simulink library "exampleMicrogridLibrary"  (R2018a)
settings: Solver=VariableStepAuto  StartTime=0.0  StopTime=10.0  RelTol=1e-3
undefined symbols (not defined in the file or in its folder): BR, D1, Delta, DiscIntNeverNeededParam, Fn, Fnom, gcbh, Ion, kv, Lithium, Ls, Rs, sps_rtmsupport, Ts, Ts_Control, Vn, Vrms
libraries: powerlib x80, simulink x29, powerlib_meascontrol x28, sps_avr x5, spsDieselMotorModel x3, electricdrivelib x2, re_lib x1
(part 2 of 5)

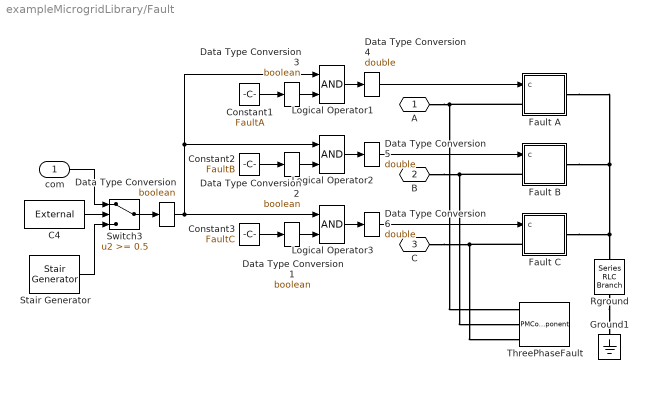
== system exampleMicrogridLibrary/Fault  ==
  com : Inport
  C4 : Constant  Value=External
  Constant1 : Constant  Value=FaultA
  Constant2 : Constant  Value=FaultB
  Constant3 : Constant  Value=FaultC
  Data Type Conversion{,1..3} (4 alike) : DataTypeConversion  OutDataTypeStr=boolean  SaturateOnIntegerOverflow=on  RndMeth=Zero
  Data Type Conversion4 : DataTypeConversion  OutDataTypeStr=double  SaturateOnIntegerOverflow=on  RndMeth=Zero
  Data Type Conversion5 : DataTypeConversion  OutDataTypeStr=double  SaturateOnIntegerOverflow=on  RndMeth=Zero
  Data Type Conversion6 : DataTypeConversion  OutDataTypeStr=double  SaturateOnIntegerOverflow=on  RndMeth=Zero
  Fault A : Subsystem  DialogController=POWERSYS.PowerSysDialog  LoadFcn=sps_rtmsupport('LoadFcn',gcbh);  StartFcn=sps_rtmsupport('StartFcn',gcbh);  StopFcn=sps_rtmsupport('StopFcn',gcbh);  mask(Breaker){InitialState=InitialStates(1)*FaultA, SwitchingTimes=[ 1/60  5/60 ], External=on, BreakerResistance=FaultResistance, SnubberResistance=SnubberResistance, SnubberCapacitance=SnubberCapacitance, Measurements=Branch current, MoreParameters=off, NoBreakLoop=off}
      mask prompts: InitialState "Initial status:"; SwitchingTimes "Switching times (s):"; BreakerResistance "Breaker resistance Ron (Ohm):"; SnubberResistance "Snubber resistance Rs (Ohm):"; SnubberCapacitance "Snubber capacitance Cs (F):"; MoreParameters "obsolete"; NoBreakLoop "Enable zero crossing detection (create an algebraic loop)"
      mask help: Implements a circuit breaker. When the external switching time option is selected, a Simulink logical signal is used to control the breaker operation.
      mask init:
      | block = gcb;
      | [WantBlockChoice,Ts,X,Y,BR,Ron] = powericon('SwitchesInit','Breaker',block,SnubberResistance,SnubberCapacitance,BreakerResistance,InitialState,SwitchingTimes,External);
      | %powericon('SetInternalModels','set',block,WantBlockChoice);
      settings: CopyFcn=sps_rtmsupport('CopyFcn',gcbh); powericon('SwitchesCopyFcn','Breaker',gcb)  DeleteFcn=sps_rtmsupport('DeleteFcn',gcbh);  UndoDeleteFcn=sps_rtmsupport('UndoDeleteFcn',gcbh);  ModelCloseFcn=sps_rtmsupport('ModelCloseFcn',gcbh);  PreSaveFcn=sps_rtmsupport('PreSaveFcn',gcbh);  PostSaveFcn=sps_rtmsupport('PostSaveFcn',gcbh);  NameChangeFcn=sps_rtmsupport('NameChangeFcn',gcbh);  PreCopyFcn=sps_rtmsupport('PreCopyFcn',gcbh);  OpenFcn=sps_rtmsupport('OpenFcn',gcbh, [3 7 8 9]);  CloseFcn=sps_rtmsupport('CloseFcn',gcbh);  PreDeleteFcn=sps_rtmsupport('PreDeleteFcn',gcbh);
      mask Help: helpview(psbhelp);
      mask Callback External: powericon('BreakerCback',gcb);
      mask Callback BreakerResistance: powericon('SwitchesEnables',gcb,'Breaker');
      mask TypeOptions Measurements: None | Branch voltage | Branch current | Branch voltage and current
      mask Display: % plot(X.p1,Y.p1,X.p2,Y.p2,X.p3,Y.p3,X.p4,Y.p4,X.p5,Y.p5,X.p6,Y.p6)
  Fault B : Subsystem  DialogController=POWERSYS.PowerSysDialog  LoadFcn=sps_rtmsupport('LoadFcn',gcbh);  StartFcn=sps_rtmsupport('StartFcn',gcbh);  StopFcn=sps_rtmsupport('StopFcn',gcbh);  mask(Breaker){InitialState=InitialStates(1)*FaultB, SwitchingTimes=[ 1/60  5/60 ], External=on, BreakerResistance=FaultResistance, SnubberResistance=SnubberResistance, SnubberCapacitance=SnubberCapacitance, Measurements=Branch current, MoreParameters=off, NoBreakLoop=off}
      mask prompts: InitialState "Initial status:"; SwitchingTimes "Switching times (s):"; BreakerResistance "Breaker resistance Ron (Ohm):"; SnubberResistance "Snubber resistance Rs (Ohm):"; SnubberCapacitance "Snubber capacitance Cs (F):"; MoreParameters "obsolete"; NoBreakLoop "Enable zero crossing detection (create an algebraic loop)"
      mask help: Implements a circuit breaker. When the external switching time option is selected, a Simulink logical signal is used to control the breaker operation.
      mask init: same as exampleMicrogridLibrary/Fault /Fault A
      settings: CopyFcn=sps_rtmsupport('CopyFcn',gcbh); powericon('SwitchesCopyFcn','Breaker',gcb)  DeleteFcn=sps_rtmsupport('DeleteFcn',gcbh);  UndoDeleteFcn=sps_rtmsupport('UndoDeleteFcn',gcbh);  ModelCloseFcn=sps_rtmsupport('ModelCloseFcn',gcbh);  PreSaveFcn=sps_rtmsupport('PreSaveFcn',gcbh);  PostSaveFcn=sps_rtmsupport('PostSaveFcn',gcbh);  NameChangeFcn=sps_rtmsupport('NameChangeFcn',gcbh);  PreCopyFcn=sps_rtmsupport('PreCopyFcn',gcbh);  OpenFcn=sps_rtmsupport('OpenFcn',gcbh, [3 7 8 9]);  CloseFcn=sps_rtmsupport('CloseFcn',gcbh);  PreDeleteFcn=sps_rtmsupport('PreDeleteFcn',gcbh);
      mask Help: helpview(psbhelp);
      mask Callback External: powericon('BreakerCback',gcb);
      mask Callback BreakerResistance: powericon('SwitchesEnables',gcb,'Breaker');
      mask TypeOptions Measurements: None | Branch voltage | Branch current | Branch voltage and current
      mask Display: % plot(X.p1,Y.p1,X.p2,Y.p2,X.p3,Y.p3,X.p4,Y.p4,X.p5,Y.p5,X.p6,Y.p6)
  Fault C : Subsystem  DialogController=POWERSYS.PowerSysDialog  LoadFcn=sps_rtmsupport('LoadFcn',gcbh);  StartFcn=sps_rtmsupport('StartFcn',gcbh);  StopFcn=sps_rtmsupport('StopFcn',gcbh);  mask(Breaker){InitialState=InitialStates(1)*FaultC, SwitchingTimes=[ 1/60  5/60 ], External=on, BreakerResistance=FaultResistance, SnubberResistance=SnubberResistance, SnubberCapacitance=SnubberCapacitance, Measurements=Branch current, MoreParameters=off, NoBreakLoop=off}
      mask prompts: InitialState "Initial status:"; SwitchingTimes "Switching times (s):"; BreakerResistance "Breaker resistance Ron (Ohm):"; SnubberResistance "Snubber resistance Rs (Ohm):"; SnubberCapacitance "Snubber capacitance Cs (F):"; MoreParameters "obsolete"; NoBreakLoop "Enable zero crossing detection (create an algebraic loop)"
      mask help: Implements a circuit breaker. When the external switching time option is selected, a Simulink logical signal is used to control the breaker operation.
      mask init: same as exampleMicrogridLibrary/Fault /Fault A
      settings: CopyFcn=sps_rtmsupport('CopyFcn',gcbh); powericon('SwitchesCopyFcn','Breaker',gcb)  DeleteFcn=sps_rtmsupport('DeleteFcn',gcbh);  UndoDeleteFcn=sps_rtmsupport('UndoDeleteFcn',gcbh);  ModelCloseFcn=sps_rtmsupport('ModelCloseFcn',gcbh);  PreSaveFcn=sps_rtmsupport('PreSaveFcn',gcbh);  PostSaveFcn=sps_rtmsupport('PostSaveFcn',gcbh);  NameChangeFcn=sps_rtmsupport('NameChangeFcn',gcbh);  PreCopyFcn=sps_rtmsupport('PreCopyFcn',gcbh);  OpenFcn=sps_rtmsupport('OpenFcn',gcbh, [3 7 8 9]);  CloseFcn=sps_rtmsupport('CloseFcn',gcbh);  PreDeleteFcn=sps_rtmsupport('PreDeleteFcn',gcbh);
      mask Help: helpview(psbhelp);
      mask Callback External: powericon('BreakerCback',gcb);
      mask Callback BreakerResistance: powericon('SwitchesEnables',gcb,'Breaker');
      mask TypeOptions Measurements: None | Branch voltage | Branch current | Branch voltage and current
      mask Display: % plot(X.p1,Y.p1,X.p2,Y.p2,X.p3,Y.p3,X.p4,Y.p4,X.p5,Y.p5,X.p6,Y.p6)
  Ground1 : powerlib/Elements/Ground  LConnTagsString=a
  Logical Operator1 : Logic
  Logical Operator2 : Logic
  Logical Operator3 : Logic
  Rground : powerlib/Elements/Series RLC Branch  LConnTagsString=__new0  RConnTagsString=__new0  BranchType=R  Resistance=GroundResistance  Inductance=0  SetiL0=off  InitialCurrent=0  Capacitance=inf  Setx0=off  InitialVoltage=0  Measurements=None
  Stair Generator : powerlib_meascontrol/Pulse & Signal Generators/Stair Generator  t=SwitchTimes  e=SwitchStatus  Ts=Ts
      settings: SourceProductName=Simscape Power Systems
  Switch3 : Switch  Threshold=0.5  ZeroCross=off  InputSameDT=on
  ThreePhaseFault : PMComponent  PhysicalDomain=powersysdomain  LeftPortType=p1  RightPortType=p1  LConnTagsString=A|B|C  mask(InnerPowersysBlock){}
  A : PMIOPort  Side=Left
  B : PMIOPort  Port=2  Side=Left
  C : PMIOPort  Port=3  Side=Left
  wires:
  Data Type Conversion6/1 -> Fault C/1(c)
  Data Type Conversion5/1 -> Fault B/1(c)
  Data Type Conversion4/1 -> Fault A/1(c)
  Logical Operator3/1 -> Data Type Conversion6/1
  Logical Operator2/1 -> Data Type Conversion5/1
  Logical Operator1/1 -> Data Type Conversion4/1
  Data Type Conversion3/1 -> Logical Operator1/2
  Constant1/1 -> Data Type Conversion3/1
  Data Type Conversion2/1 -> Logical Operator2/2
  Constant2/1 -> Data Type Conversion2/1
  Data Type Conversion1/1 -> Logical Operator3/2
  Constant3/1 -> Data Type Conversion1/1
  Data Type Conversion/1 -> Logical Operator1/1, Logical Operator2/1, Logical Operator3/1
  Switch3/1 -> Data Type Conversion/1
  C4/1 -> Switch3/2
  Stair Generator/1 -> Switch3/3
  com/1 -> Switch3/1
  connections:
  Fault B/RConn1 -- Fault A/RConn1 -- Fault C/RConn1 -- Rground/LConn1
  C/RConn1 -- Fault C/LConn1 -- ThreePhaseFault/LConn3
  B/RConn1 -- Fault B/LConn1 -- ThreePhaseFault/LConn2
  A/RConn1 -- Fault A/LConn1 -- ThreePhaseFault/LConn1
  Rground/RConn1 -- Ground1/LConn1

== system exampleMicrogridLibrary/Grid-Connected Battery (EMT with Simple Controls) ==
  PQref : Inport  SampleTime=Ts_Control
  Battery : electricdrivelib/Extra Sources/Battery  BatType=Lithium-Ion  ShowTempParam=off  ThermalPreset=no  ShowAgeParam=off  NomV=Vnom_dc  NomQ=Bcap  SOC=75  Batt_Tr=30  PresetModel=on  MaxQ=500  MinV=360  FullV=558.7138  Dis_rate=217.3913  R=0.0096  Normal_OP=452.1739  expZone="[518.5852      24.56522]"  current=[6.5 13 32.5]  Units=Time  Tci=20  NomT=25  T2=0  MaxQ2=2.208  FullV2=3.45  Normal_OP2=2.8  expZone2="[3.22        0.23]"  Rca=0.6  ti=1000  Dp=0  Neq0=0  Tsim=1e6  Ta1=25  Qeol=5.4*0.9  Reol=0.013333*1.2  Char_age=[2.3478, 3]  Dis_age=[2.3478, 10]  N1=1500  N2=10500  N3=1000  N4=1400  Ta2=45  N5=950
  Battery Controller : Subsystem  SystemSampleTime=Ts
  Bus Selector : BusSelector  OutputSignals=Vabc,Iabc
  DC Link : Subsystem
  Grid Inverter : Subsystem
  Inverter Control : Subsystem
  Measures : Subsystem
  Rate Transition2 : RateTransition  OutPortSampleTime=Ts_Control
  A : PMIOPort  Side=Right
  B : PMIOPort  Port=2  Side=Right
  C : PMIOPort  Port=3  Side=Right
  m : Outport
  wires:
  PQref/1 -> Battery Controller/2(PQref)
  Rate Transition2/1 -> Battery Controller/1(m), Bus Selector/1
  Inverter Control/1(Uref) -> Grid Inverter/1(Uref)
  Bus Selector/1 -> Inverter Control/1(Vabc_prim)  "<Vabc>"
  Bus Selector/2 -> Inverter Control/2(Iabc_prim)  "<Iabc>"
  Grid Inverter/1(m) -> [m_inv]
  [m_inv] -> Measures/1(Grid)
  [m_batt] -> Measures/2(Battery)
  Measures/1(m) -> m/1
  Battery/1 -> [m_batt]
  [m_inv] -> Rate Transition2/1
  Battery Controller/1(Idq_ref) -> Inverter Control/3(Idq_ref)
  connections:
  Battery/LConn1 -- DC Link/LConn1
  Battery/LConn2 -- DC Link/LConn2
  Grid Inverter/LConn3 -- DC Link/RConn3
  A/RConn1 -- Grid Inverter/RConn1
  B/RConn1 -- Grid Inverter/RConn2
  C/RConn1 -- Grid Inverter/RConn3
  Grid Inverter/LConn1 -- DC Link/RConn1
  DC Link/RConn2 -- Grid Inverter/LConn2

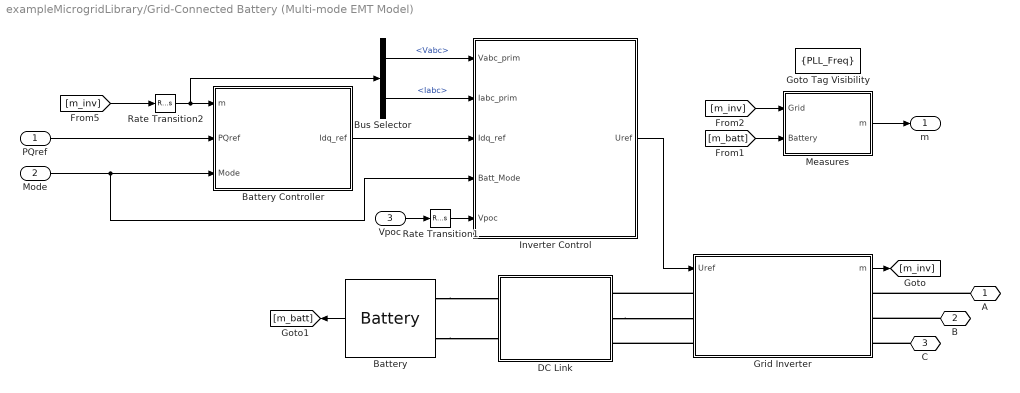
== system exampleMicrogridLibrary/Grid-Connected Battery (Multi-mode EMT Model) ==
  PQref : Inport  SampleTime=Ts_Control
  Mode : Inport  Port=2
  Vpoc : Inport  Port=3
  Battery : electricdrivelib/Extra Sources/Battery  BatType=Lithium-Ion  ShowTempParam=off  ThermalPreset=no  ShowAgeParam=off  NomV=Vnom_dc  NomQ=Bcap  SOC=75  Batt_Tr=30  PresetModel=on  MaxQ=500  MinV=360  FullV=558.7138  Dis_rate=217.3913  R=0.0096  Normal_OP=452.1739  expZone="[518.5852      24.56522]"  current=[6.5 13 32.5]  Units=Time  Tci=20  NomT=25  T2=0  MaxQ2=2.208  FullV2=3.45  Normal_OP2=2.8  expZone2="[3.22        0.23]"  Rca=0.6  ti=1000  Dp=0  Neq0=0  Tsim=1e6  Ta1=25  Qeol=5.4*0.9  Reol=0.013333*1.2  Char_age=[2.3478, 3]  Dis_age=[2.3478, 10]  N1=1500  N2=10500  N3=1000  N4=1400  Ta2=45  N5=950
  Battery Controller : Subsystem  SystemSampleTime=Ts
  Bus Selector : BusSelector  OutputSignals=Vabc,Iabc
  DC Link : Subsystem
  Goto Tag Visibility : GotoTagVisibility  GotoTag=PLL_Freq
  Grid Inverter : Subsystem
  Inverter Control : Subsystem
  Measures : Subsystem
  Rate Transition1 : RateTransition  OutPortSampleTime=Ts_Control
  Rate Transition2 : RateTransition  OutPortSampleTime=Ts_Control
  A : PMIOPort  Side=Right
  B : PMIOPort  Port=2  Side=Right
  C : PMIOPort  Port=3  Side=Right
  m : Outport
  wires:
  Battery Controller/1(Idq_ref) -> Inverter Control/3(Idq_ref)
  [m_inv] -> Rate Transition2/1
  Battery/1 -> [m_batt]
  Measures/1(m) -> m/1
  [m_batt] -> Measures/2(Battery)
  [m_inv] -> Measures/1(Grid)
  Grid Inverter/1(m) -> [m_inv]
  Bus Selector/2 -> Inverter Control/2(Iabc_prim)  "<Iabc>"
  Bus Selector/1 -> Inverter Control/1(Vabc_prim)  "<Vabc>"
  Inverter Control/1(Uref) -> Grid Inverter/1(Uref)
  Rate Transition2/1 -> Battery Controller/1(m), Bus Selector/1
  PQref/1 -> Battery Controller/2(PQref)
  Mode/1 -> Battery Controller/3(Mode), Inverter Control/4(Batt_Mode)
  Vpoc/1 -> Rate Transition1/1
  Rate Transition1/1 -> Inverter Control/5(Vpoc)
  connections:
  DC Link/RConn2 -- Grid Inverter/LConn2
  Grid Inverter/LConn1 -- DC Link/RConn1
  C/RConn1 -- Grid Inverter/RConn3
  B/RConn1 -- Grid Inverter/RConn2
  A/RConn1 -- Grid Inverter/RConn1
  Grid Inverter/LConn3 -- DC Link/RConn3
  Battery/LConn2 -- DC Link/LConn2
  Battery/LConn1 -- DC Link/LConn1

== system exampleMicrogridLibrary/Ideal Source ==
  Vm : Inport
  Freq : Inport  Port=2
  Bias1 : Bias  Bias=-2*pi/3
  Bias2 : Bias  Bias=2*pi/3
  Gain4 : Gain  Gain=1/sqrt(3)*sqrt(2)
  Magnitude-Angle to Complex_A : MagnitudeAngleToComplex
  Magnitude-Angle to Complex_B : MagnitudeAngleToComplex
  Magnitude-Angle to Complex_C : MagnitudeAngleToComplex
  Mux : Mux  Inputs=3
  Subsystem : Subsystem
  ThreePhaseSourceBlk : PMComponent  PhysicalDomain=powersysdomain  LeftPortType=p1  RightPortType=p1  LConnTagsString=N  RConnTagsString=A|B|C  mask(InnerPowersysBlock){}
      mask Display: disp('SPS internal use\nDo not delete')
  A : PMIOPort  Side=Right
  B : PMIOPort  Port=2  Side=Right
  C : PMIOPort  Port=3  Side=Right
  tag scope: T96_8972_14978298618803=global
  wires:
  Mux/1 -> [T96_8972_14978298618803]
  Bias1/1 -> Magnitude-Angle to Complex_B/2
  Magnitude-Angle to Complex_C/1 -> Mux/3
  Bias2/1 -> Magnitude-Angle to Complex_C/2
  Magnitude-Angle to Complex_B/1 -> Mux/2
  Subsystem/1(Phase) -> Magnitude-Angle to Complex_A/2, Bias1/1, Bias2/1
  Vm/1 -> Gain4/1
  Magnitude-Angle to Complex_A/1 -> Mux/1
  Gain4/1 -> Magnitude-Angle to Complex_A/1, Magnitude-Angle to Complex_C/1, Magnitude-Angle to Complex_B/1
  Freq/1 -> Subsystem/1(Freq (Hz))
  connections:
  A/RConn1 -- ThreePhaseSourceBlk/RConn1
  B/RConn1 -- ThreePhaseSourceBlk/RConn2
  C/RConn1 -- ThreePhaseSourceBlk/RConn3

== system exampleMicrogridLibrary/Line (PI) ==
  A : PMIOPort  Side=Left
  a : PMIOPort  Port=2  Side=Right
  B : PMIOPort  Port=3  Side=Left
  b : PMIOPort  Port=4  Side=Right
  C : PMIOPort  Port=5  Side=Left
  c : PMIOPort  Port=6  Side=Right
  connections:
  C/RConn1 -- c/RConn1
  B/RConn1 -- b/RConn1
  A/RConn1 -- a/RConn1

== system exampleMicrogridLibrary/Line (Series) ==
  Series Impedance : powerlib/Elements/Three-Phase Series RLC Branch  LConnTagsString=A|B|C  RConnTagsString=A|B|C  BranchType=RL  Resistance=R0*Length  Inductance=L0*Length  Capacitance=0  Measurements=None
  A : PMIOPort  Side=Left
  a : PMIOPort  Port=2  Side=Right
  B : PMIOPort  Port=3  Side=Left
  b : PMIOPort  Port=4  Side=Right
  C : PMIOPort  Port=5  Side=Left
  c : PMIOPort  Port=6  Side=Right
  connections:
  Series Impedance/LConn3 -- c/RConn1
  Series Impedance/LConn2 -- b/RConn1
  Series Impedance/LConn1 -- a/RConn1
  C/RConn1 -- Series Impedance/RConn3
  B/RConn1 -- Series Impedance/RConn2
  A/RConn1 -- Series Impedance/RConn1

== system exampleMicrogridLibrary/Power Equation Wind Turbine (PQ Model) ==
  Wind (m/s) : Inport
  Qref (pu) : Inport  Port=2
  Active Power Dynamics : Subsystem  VariantControl=T6NotZero
      mask Display: disp('1 / (1 + s T_P)','texmode','on');
  Ground : powerlib/Elements/Ground  LConnTagsString=a
  Mux : Mux  Inputs=2
  Reactive Power Dynamics : Subsystem  VariantControl=T6NotZero
      mask Display: disp('1 / (1 + s T_Q)','texmode','on');
  Saturation : Saturate  UpperLimit=Qmax  LowerLimit=-Qmax
  Shunt (Numerical Stability) : powerlib/Elements/Three-Phase Series RLC Branch  LConnTagsString=A|B|C  RConnTagsString=A|B|C  BranchType=R  Resistance=1e9  Inductance=1e-3  Capacitance=1e-6  Measurements=None
  Three-Phase Dynamic Load : powerlib/Elements/Three-Phase Dynamic Load  NominalVoltage=[Vrms Fnom]  ActiveReactivePowers=[50e6 25e6]  PositiveSequence=[0.994 -11.8]  ExternalControl=on  NpNq=[1.3 2]  TimeConstants="[0  0  0  0]"  MinimumVoltage=0.7  Tfilter=1e-4  LoadFlowParameters=[4,0,0,0,0]
      settings: SourceProductName=Simscape Power Systems  SourceProductBaseCode=PS
  Wind Turbine Power Equation : Subsystem
  A : PMIOPort  Side=Left
  B : PMIOPort  Port=2  Side=Left
  C : PMIOPort  Port=3  Side=Left
  m : Outport
  wires:
  Three-Phase Dynamic Load/1 -> m/1
  Wind (m/s)/1 -> Wind Turbine Power Equation/1(Wind (m/s))
  Wind Turbine Power Equation/1(Pwind) -> Active Power Dynamics/1(In)
  Mux/1 -> Three-Phase Dynamic Load/1
  Active Power Dynamics/1(Out) -> Mux/1
  Reactive Power Dynamics/1(Out) -> Mux/2
  Saturation/1 -> Reactive Power Dynamics/1(In)
  Qref (pu)/1 -> Saturation/1
  connections:
  B/RConn1 -- Three-Phase Dynamic Load/LConn2 -- Shunt (Numerical Stability)/LConn2
  C/RConn1 -- Three-Phase Dynamic Load/LConn3 -- Shunt (Numerical Stability)/LConn3
  A/RConn1 -- Three-Phase Dynamic Load/LConn1 -- Shunt (Numerical Stability)/LConn1
  Shunt (Numerical Stability)/RConn3 -- Shunt (Numerical Stability)/RConn2 -- Shunt (Numerical Stability)/RConn1 -- Ground/LConn1

== system exampleMicrogridLibrary/Relay ==
  Input : Inport
  " Shunt (Numerical Stability)" : powerlib/Elements/Three-Phase Series RLC Branch  LConnTagsString=A|B|C  RConnTagsString=A|B|C  BranchType=R  Resistance=1e7  Inductance=1e-3  Capacitance=1e-6  Measurements=None
  Breaker (Pure Discrete) : Subsystem  Commented=on  DialogController=POWERSYS.PowerSysDialog  LoadFcn=sps_rtmsupport('LoadFcn',gcbh);  StartFcn=sps_rtmsupport('StartFcn',gcbh);  StopFcn=sps_rtmsupport('StopFcn',gcbh);  mask(Three-Phase Breaker){InitialState=closed, SwitchA=on, SwitchB=on, SwitchC=on, SwitchTimes=2/60, External=on, BreakerResistance=1e-4, SnubberResistance=1e15, SnubberCapacitance=inf, Measurements=None}
      mask prompts: InitialState "Initial status:"; SwitchA "Phase A"; SwitchB "Phase B"; SwitchC "Phase C"; SwitchTimes "Switching times (s):"; BreakerResistance "Breaker resistance Ron (Ohm):"; SnubberResistance "Snubber resistance Rs (Ohm):"; SnubberCapacitance "Snubber capacitance Cs (F):"
      mask help: Implements a three-phase circuit breaker. When the external switching time mode is selected, a Simulink logical signal is used to control the breaker operation.
      mask init:
      | block = gcb;
      | [X,Y,SwitchStatus,InitialState,Ts,Switch_Times] = powericon('ThreePhaseBreakerInit',block,InitialState,SwitchTimes,External,SnubberResistance,SnubberCapacitance);
      | powericon('ThreePhaseBreakerCback',block);
      settings: CopyFcn=sps_rtmsupport('CopyFcn',gcbh);  DeleteFcn=sps_rtmsupport('DeleteFcn',gcbh);  UndoDeleteFcn=sps_rtmsupport('UndoDeleteFcn',gcbh);  ModelCloseFcn=sps_rtmsupport('ModelCloseFcn',gcbh);  PreSaveFcn=sps_rtmsupport('PreSaveFcn',gcbh);  PostSaveFcn=sps_rtmsupport('PostSaveFcn',gcbh);  NameChangeFcn=sps_rtmsupport('NameChangeFcn',gcbh);  PreCopyFcn=sps_rtmsupport('PreCopyFcn',gcbh);  OpenFcn=sps_rtmsupport('OpenFcn',gcbh, [1 2 3 4 6 10]);  CloseFcn=sps_rtmsupport('CloseFcn',gcbh);  PreDeleteFcn=sps_rtmsupport('PreDeleteFcn',gcbh);
      mask Help: helpview(psbhelp)
      mask TypeOptions InitialState: open | closed
      mask Callback External: powericon('ThreePhaseBreakerCback',gcb);
      mask TypeOptions Measurements: None | Breaker voltages | Breaker currents | Breaker voltages and currents
      mask DialogControl Container3 Prompt: Switching of:
      mask Display: plot(X.p1,Y.p1,X.p2,Y.p2,X.p3,Y.p3,X.p4,Y.p4,X.p5,Y.p5,X.p6,Y.p6)
  Breaker (SPS Default) : powerlib/Elements/Three-Phase Breaker  InitialState=closed  SwitchA=on  SwitchB=on  SwitchC=on  SwitchTimes="[1/60  5/60]"  External=on  BreakerResistance=1e-4  SnubberResistance=1e15  SnubberCapacitance=inf  Measurements=None
  Ground : powerlib/Elements/Ground  LConnTagsString=a
  Ground1 : powerlib/Elements/Ground  LConnTagsString=a
  Ground2 : Ground
  Shunt (Numerical Stability) : powerlib/Elements/Three-Phase Series RLC Branch  LConnTagsString=A|B|C  RConnTagsString=A|B|C  BranchType=R  Resistance=1e7  Inductance=1e-3  Capacitance=1e-6  Measurements=None
  A : PMIOPort  Tag=PMCPort  Side=Left
  B : PMIOPort  Tag=PMCPort  Port=2  Side=Left
  C : PMIOPort  Tag=PMCPort  Port=3  Side=Left
  a : PMIOPort  Tag=PMCPort  Port=4  Side=Right
  b : PMIOPort  Tag=PMCPort  Port=5  Side=Right
  c : PMIOPort  Tag=PMCPort  Port=6  Side=Right
  m : Outport
  wires:
  Ground2/1 -> m/1
  Input/1 -> Breaker (SPS Default)/1
  connections:
  C/RConn1 -- Breaker (SPS Default)/LConn3 -- Shunt (Numerical Stability)/LConn3
  a/RConn1 -- Breaker (SPS Default)/RConn1 -- " Shunt (Numerical Stability)"/LConn1
  b/RConn1 -- Breaker (SPS Default)/RConn2 -- " Shunt (Numerical Stability)"/LConn2
  " Shunt (Numerical Stability)"/RConn2 -- " Shunt (Numerical Stability)"/RConn1 -- Ground1/LConn1 -- " Shunt (Numerical Stability)"/RConn3
  c/RConn1 -- Breaker (SPS Default)/RConn3 -- " Shunt (Numerical Stability)"/LConn3
  B/RConn1 -- Breaker (SPS Default)/LConn2 -- Shunt (Numerical Stability)/LConn2
  A/RConn1 -- Breaker (SPS Default)/LConn1 -- Shunt (Numerical Stability)/LConn1
  Shunt (Numerical Stability)/RConn1 -- Shunt (Numerical Stability)/RConn2 -- Ground/LConn1 -- Shunt (Numerical Stability)/RConn3

== system exampleMicrogridLibrary/SPS-Simulink Interface ==
  Vin : Inport
  EMT : Subsystem  VariantControl=EMT
  Phasor : Subsystem  VariantControl=Phasor
  A : PMIOPort  Side=Right
  B : PMIOPort  Port=2  Side=Right
  C : PMIOPort  Port=3  Side=Right
  Vout : Outport

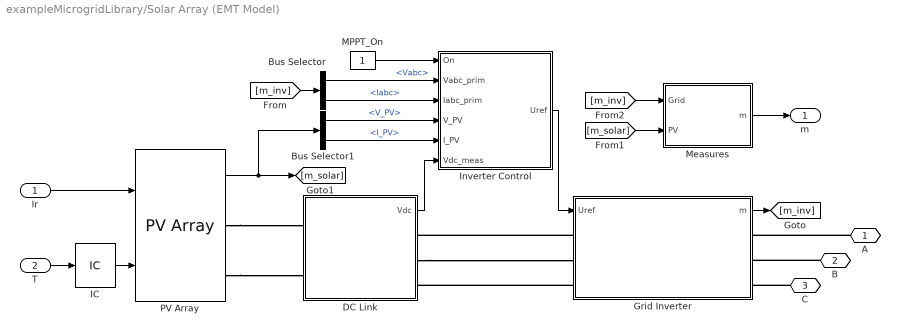
== system exampleMicrogridLibrary/Solar Array (EMT Model) ==
  Ir : Inport
  T : Inport  Port=2
  Bus Selector : BusSelector  OutputSignals=Vabc,Iabc
  Bus Selector1 : BusSelector  OutputSignals=V_PV,I_PV
  DC Link : Subsystem
  Grid Inverter : Subsystem
  IC : InitialCondition  Value=45
  Inverter Control : Subsystem
  MPPT_On : Constant
  Measures : Subsystem
  PV Array : re_lib/Solar/PV Array  Npar=round(35*Pmod)  Nser=7  PlotType=array @ 1000 W/m2 & specified temperatures  S_vec="[ 1000  500  100 ]"  Temp_C_vec="[ 45 25  ]"  ModuleName=SunPower SPR-415E-WHT-D  PlotWhenSelected=off  Pm=414.801  Ncell=128  Voc=85.3  Isc=6.09  Vm=72.9  Im=5.69  beta_Voc_pc=-0.229  alpha_Isc_pc=0.030706  beta_Voc=-0.19534  alpha_Isc=0.00187  IL=6.0978  I0=7.1712e-13  nI=0.87223  Rsh=419.7813  Rs=0.5371  BAL=on  Tc=1e-6  Tfilter=5e-5
      settings: AttributesFormatString=|
      | %<ModuleName>
      | %<Nser>-module string
      | %<Npar> parallel strings
  A : PMIOPort  Side=Right
  B : PMIOPort  Port=2  Side=Right
  C : PMIOPort  Port=3  Side=Right
  m : Outport
  wires:
  Measures/1(m) -> m/1
  [m_solar] -> Measures/2(PV)
  [m_inv] -> Measures/1(Grid)
  IC/1 -> PV Array/2
  PV Array/1 -> Bus Selector1/1, [m_solar]
  DC Link/1(Vdc) -> Inverter Control/6(Vdc_meas)
  [m_inv] -> Bus Selector/1
  Grid Inverter/1(m) -> [m_inv]
  T/1 -> IC/1
  MPPT_On/1 -> Inverter Control/1(On)
  Bus Selector/2 -> Inverter Control/3(Iabc_prim)  "<Iabc>"
  Bus Selector/1 -> Inverter Control/2(Vabc_prim)  "<Vabc>"
  Bus Selector1/2 -> Inverter Control/5(I_PV)  "<I_PV>"
  Bus Selector1/1 -> Inverter Control/4(V_PV)  "<V_PV>"
  Inverter Control/1(Uref) -> Grid Inverter/1(Uref)
  Ir/1 -> PV Array/1
  connections:
  DC Link/RConn2 -- Grid Inverter/LConn2
  Grid Inverter/LConn1 -- DC Link/RConn1
  C/RConn1 -- Grid Inverter/RConn3
  B/RConn1 -- Grid Inverter/RConn2
  A/RConn1 -- Grid Inverter/RConn1
  Grid Inverter/LConn3 -- DC Link/RConn3
  PV Array/RConn2 -- DC Link/LConn2
  PV Array/RConn1 -- DC Link/LConn1

== system exampleMicrogridLibrary/Solar Array (PQ Model) ==
  P : Inport
  Bus Selector : BusSelector  OutputSignals=Active power P (W)
  Constant11 : Constant  Value=0
  Mux1 : Mux  Inputs=2
  Simple Solar Inverter : powerlib/Elements/Three-Phase Dynamic Load  NominalVoltage=[Vn Fn]  ActiveReactivePowers=[-250000 -3.38813e-13]  PositiveSequence=[0.999844 -0.0038635]  ExternalControl=on  NpNq=[1.3 2]  TimeConstants="[0  0  0  0]"  MinimumVoltage=0.7  Tfilter=1e-2  LoadFlowParameters=[4,0,0,0,0]
      settings: SourceProductName=Simscape Power Systems  SourceProductBaseCode=PS
  Unary Minus : UnaryMinus
  Unary Minus1 : UnaryMinus
  A : PMIOPort  Side=Right
  B : PMIOPort  Port=2  Side=Right
  C : PMIOPort  Port=3  Side=Right
  m : Outport
  wires:
  P/1 -> Unary Minus/1
  Unary Minus/1 -> Mux1/1
  Mux1/1 -> Simple Solar Inverter/1
  Constant11/1 -> Mux1/2
  Simple Solar Inverter/1 -> Bus Selector/1
  Bus Selector/1 -> Unary Minus1/1  "<Active power P (W)>"
  Unary Minus1/1 -> m/1
  connections:
  Simple Solar Inverter/LConn2 -- B/RConn1
  Simple Solar Inverter/LConn3 -- C/RConn1
  Simple Solar Inverter/LConn1 -- A/RConn1

== system exampleMicrogridLibrary/Transformer ==
  Ground : powerlib/Elements/Ground  LConnTagsString=a
  Shunt (Numerical Stability) : powerlib/Elements/Three-Phase Series RLC Branch  LConnTagsString=A|B|C  RConnTagsString=A|B|C  BranchType=R  Resistance=1e7  Inductance=1e-3  Capacitance=1e-6  Measurements=None
  Three-Phase Transformer (Two Windings) : powerlib/Elements/Three-Phase Transformer (Two Windings)  Winding1Connection=Delta (D1)  Winding2Connection=Yg  CoreType=Three single-phase transformers  SetSaturation=off  Hysteresis=off  DataFile='hysteresis'  SetInitialFlux=off  Measurements=None  UNITS=pu  NominalPower=[S Freq]  Winding1=[Vp 0 0]  Winding2=[Vs Z/Ratio Z/(2*pi*Freq)]  Rm=500  Lm=500  L0=0.5  Saturation=[ 0,0 ; 0.0024,1.2 ; 1.0,1.52 ]  InitialFluxes=[ 0.8 , -0.8 , 0.7 ]  MoreParameters=off  BreakLoop=off  DataType=off  TransfoNumber=1
  A : PMIOPort  Tag=PMCPort  Side=Left
  B : PMIOPort  Tag=PMCPort  Port=2  Side=Left
  C : PMIOPort  Tag=PMCPort  Port=3  Side=Left
  a : PMIOPort  Tag=PMCPort  Port=4  Side=Right
  b : PMIOPort  Tag=PMCPort  Port=5  Side=Right
  c : PMIOPort  Tag=PMCPort  Port=6  Side=Right
  connections:
  a/RConn1 -- Three-Phase Transformer (Two Windings)/RConn1
  b/RConn1 -- Three-Phase Transformer (Two Windings)/RConn2
  c/RConn1 -- Three-Phase Transformer (Two Windings)/RConn3
  A/RConn1 -- Shunt (Numerical Stability)/LConn1 -- Three-Phase Transformer (Two Windings)/LConn1
  B/RConn1 -- Shunt (Numerical Stability)/LConn2 -- Three-Phase Transformer (Two Windings)/LConn2
  Three-Phase Transformer (Two Windings)/LConn3 -- Shunt (Numerical Stability)/LConn3 -- C/RConn1
  Shunt (Numerical Stability)/RConn1 -- Shunt (Numerical Stability)/RConn2 -- Ground/LConn1 -- Shunt (Numerical Stability)/RConn3

== system exampleMicrogridLibrary/Variable Load ==
  Load : Inport
  Dynamic Load Control : Subsystem
  Simple Three-Phase Load : powerlib/Elements/Three-Phase Dynamic Load  NominalVoltage=[Vn Fn]  ActiveReactivePowers=[200000 45883.1]  PositiveSequence=[0.999844 -0.0038635]  ExternalControl=on  NpNq=[1.3 2]  TimeConstants="[0  0  0  0]"  MinimumVoltage=0.7  Tfilter=1e-2  LoadFlowParameters=[4,0,0,0,0]
      settings: SourceProductName=Simscape Power Systems  SourceProductBaseCode=PS
  Terminator : Terminator
  A : PMIOPort  Side=Right
  B : PMIOPort  Port=2  Side=Right
  C : PMIOPort  Port=3  Side=Right
  wires:
  Simple Three-Phase Load/1 -> Terminator/1
  Load/1 -> Dynamic Load Control/1(P0)
  Dynamic Load Control/1(PQ) -> Simple Three-Phase Load/1
  connections:
  Simple Three-Phase Load/LConn1 -- A/RConn1
  Simple Three-Phase Load/LConn3 -- C/RConn1
  Simple Three-Phase Load/LConn2 -- B/RConn1

== system exampleMicrogridLibrary/Diesel Generator (Full Genset Controls)/Continuous ==
  Mode : Inport
  PQwv_ref : Inport  Port=2
  Automatic Generator Controls : Subsystem
  Diesel Engine Governor : spsDieselMotorModel/Diesel Engine Governor  K=29  Tr=[0.01 0.02 0.2]  Ta=[0.25 0.009 0.0384]  Tlim=[0 1.1]  Td=0.024  Pm0=0.80192
  Excitation System : sps_avr/AC1A Excitation System  Tr=20e-3  KaTa=[400 0.02]  VAminmax=[-14.5 14.5]  VRminmax=[-5.43 6.03]  KfTf=[0.03 1.0]  TbTc=[0 0]  KeTe=[1.0 0.80]  Ve12=[4.18 3.14]  SeVe12=[0.10 0.03]  Kd=0.38  Kc=0.20  v0=[1 1.3069]  TsBlock=0
      settings: SourceProductName=Simscape Power Systems  SourceProductBaseCode=PS
  Generator Measures : Subsystem
  Ground : Ground
  Selected Measurements : Subsystem
  Shunt : powerlib/Elements/Three-Phase Parallel RLC Load  LConnTagsString=A|B|C  Configuration=Y (grounded)  NominalVoltage=Vn  Vabc=[1e3 1e3 1e3]  Vabcp=[1e3 1e3 1e3]  NominalFrequency=Fn  UnbalancedPower=off  ActivePower=Pn*0.05  InductivePower=0  CapacitivePower=0  Pabc=[10e3 9e3 11e3]  QLabc=[100 90 110]  QCabc=[100 90 110]  Pabcp=[10e3 9e3 11e3]  QLabcp=[100 90 110]  QCabcp=[100 90 110]  Measurements=None  LoadType=constant Z
  Synchronous Machine : powerlib/Machines/Synchronous Machine pu Standard  PresetModel=No  MechanicalLoad=Mechanical power Pm  ShowDetailedParameters=on  RotorType=Salient-pole  Units=per unit standard parameters  MeasurementBus=off  NominalParameters=[ Pn Vn Fn]  Reactances1=[ 1.81, 0.3, 0.23, 1.76, 0.65, 0.25, 0.15 ]  Reactances2="[ 1.305, 0.296, 0.252, 0.474,  0.243,  0.18 ]"  dAxisTimeConstants=Open-circuit  qAxisTimeConstants=Short-circuit  TimeConstants1="[ 4.4849  0.0681  0.1  ]"  TimeConstants2=[ 8.0, 0.03, 1.0, 0.07 ]  TimeConstants3="[  4.49  0.0681  0.0513  ]"  TimeConstants4=[ 8.0, 0.03, 0.3371, 0.0295 ]  TimeConstants5=[ 1.01, 0.053, 0.1 ]  TimeConstants6=[ 1.3201, 0.023, 1.0, 0.07 ]  TimeConstants7=[0.012 0.003 0.003]  TimeConstants8=[ 1.3201, 0.0231, 0.3371, 0.0295 ]  StatorResistance=0.003  Mechanical=[3.7 0 1 ]  PolePairs=20  InitialConditions=[0 -69.2788 0.8 0.8 0.8 0 -120 120 1.30695]  SetSaturation=off  Saturation=[0.6404,0.7127,0.8441,0.9214,0.9956,1.082,1.19,1.316,1.457;0.7,0.7698,0.8872,0.9466,0.9969,1.046,1.1,1.151,1.201]  LoadFlowParameters=[1,0,0,0,0]  TsPowergui=0  TsBlock=-1  IterativeModel=Trapezoidal non iterative  IterativeDiscreteModel=Trapezoidal non iterative  BusType=PQ  Pref=Pn*P0  Qref=0  Qmin=-inf  Qmax=inf  PLF=0  QLF=0
      settings: SourceProductName=Simscape Power Systems
  A : PMIOPort  Side=Right
  B : PMIOPort  Port=2  Side=Right
  C : PMIOPort  Port=3  Side=Right
  m : Outport
  wires:
  Generator Measures/2(Vt) -> Excitation System/2
  Excitation System/1 -> Synchronous Machine/2
  Automatic Generator Controls/1(wref) -> Diesel Engine Governor/1
  Diesel Engine Governor/1 -> Synchronous Machine/1
  Generator Measures/1(Ifd) -> Excitation System/3
  Ground/1 -> Excitation System/4
  Synchronous Machine/1 -> Selected Measurements/1(m), Generator Measures/1(m)
  Selected Measurements/1(sm) -> [GenM], m/1
  Automatic Generator Controls/2(vref) -> Excitation System/1
  Generator Measures/3(wm) -> Diesel Engine Governor/2
  [GenM] -> Automatic Generator Controls/3(GenM)
  Mode/1 -> Automatic Generator Controls/1(Mode)
  PQwv_ref/1 -> Automatic Generator Controls/2(PQwv_ref)
  connections:
  B/RConn1 -- Shunt/LConn2 -- Synchronous Machine/RConn2
  Shunt/LConn3 -- C/RConn1 -- Synchronous Machine/RConn3
  Shunt/LConn1 -- A/RConn1 -- Synchronous Machine/RConn1

== system exampleMicrogridLibrary/Diesel Generator (Full Genset Controls)/Discrete ==
  Mode : Inport
  PQwv_ref : Inport  Port=2
  Automatic Generator Controls : Subsystem
  Diesel Engine Governor : Subsystem  mask(Diesel Engine & Governor){K=29, Tr=[0.01 0.02 0.2], Ta=[0.25 0.009 0.0384], Tlim=[0 1.1], Td=0.024, Pm0=0.80192, Ts=Ts}
      mask prompts: K "Regulator gain K:"; Tr "Regulator time constants [T1 T2 T3 ] (s) :"; Ta "Actuator time constants [T4 T5 T6] (s) :"; Tlim "Torque limits [Tmin Tmax] (pu) :"; Td "Engine time delay Td (s) :"; Pm0 "Initial value of mechanical power  Pm0 (pu) :"; Ts "Sample Time (s)"
      mask help:
      | This block implements a diesel engine and governor system:
      | 1st and 2nd inputs: Desired and actual speed (pu)
      | Output: Diesel engine mechanical power.Motor inertia should be combined with generator.
      | Controller transfer function:
      |      Hc=K.(1+T3.s)/(1+T1.s+T1.T2.s^2)
      | Actuator transfer function :
      |      Ha= (1+T4.s) / [ (s (1+T5.s)(1+T6.s) ]
      | Motor :
      |      Time delay Td
      |
      | (See reference in Tutorial Session 5)
  Excitation System : sps_avr/AC1A Excitation System  Tr=20e-3  KaTa=[400 0.02]  VAminmax=[-14.5 14.5]  VRminmax=[-5.43 6.03]  KfTf=[0.03 1.0]  TbTc=[0 0]  KeTe=[1.0 0.80]  Ve12=[4.18 3.14]  SeVe12=[0.10 0.03]  Kd=0.38  Kc=0.20  v0=[1 1.3069]  TsBlock=Ts
      settings: SourceProductName=Simscape Power Systems  SourceProductBaseCode=PS
  Generator Measures : Subsystem
  Ground : Ground
  Selected Measurements : Subsystem
  Shunt : powerlib/Elements/Three-Phase Parallel RLC Load  LConnTagsString=A|B|C  Configuration=Y (grounded)  NominalVoltage=Vn  Vabc=[1e3 1e3 1e3]  Vabcp=[1e3 1e3 1e3]  NominalFrequency=Fn  UnbalancedPower=off  ActivePower=Pn*0.05  InductivePower=0  CapacitivePower=0  Pabc=[10e3 9e3 11e3]  QLabc=[100 90 110]  QCabc=[100 90 110]  Pabcp=[10e3 9e3 11e3]  QLabcp=[100 90 110]  QCabcp=[100 90 110]  Measurements=None  LoadType=constant Z
  Synchronous Machine : powerlib/Machines/Synchronous Machine pu Standard  PresetModel=No  MechanicalLoad=Mechanical power Pm  ShowDetailedParameters=on  RotorType=Salient-pole  Units=per unit standard parameters  MeasurementBus=off  NominalParameters=[ Pn Vn Fn]  Reactances1=[ 1.81, 0.3, 0.23, 1.76, 0.65, 0.25, 0.15 ]  Reactances2="[ 1.305, 0.296, 0.252, 0.474,  0.243,  0.18 ]"  dAxisTimeConstants=Open-circuit  qAxisTimeConstants=Short-circuit  TimeConstants1="[ 4.4849  0.0681  0.1  ]"  TimeConstants2=[ 8.0, 0.03, 1.0, 0.07 ]  TimeConstants3="[  4.49  0.0681  0.0513  ]"  TimeConstants4=[ 8.0, 0.03, 0.3371, 0.0295 ]  TimeConstants5=[ 1.01, 0.053, 0.1 ]  TimeConstants6=[ 1.3201, 0.023, 1.0, 0.07 ]  TimeConstants7=[0.012 0.003 0.003]  TimeConstants8=[ 1.3201, 0.0231, 0.3371, 0.0295 ]  StatorResistance=0.003  Mechanical=[3.7 0 1 ]  PolePairs=20  InitialConditions=[0 -69.2788 0.8 0.8 0.8 0 -120 120 1.30695]  SetSaturation=off  Saturation=[0.6404,0.7127,0.8441,0.9214,0.9956,1.082,1.19,1.316,1.457;0.7,0.7698,0.8872,0.9466,0.9969,1.046,1.1,1.151,1.201]  LoadFlowParameters=[1,0,0,0,0]  TsPowergui=0  TsBlock=Ts  IterativeModel=Trapezoidal non iterative  IterativeDiscreteModel=Trapezoidal non iterative  BusType=PQ  Pref=Pn*P0  Qref=0  Qmin=-inf  Qmax=inf  PLF=0  QLF=0
      settings: SourceProductName=Simscape Power Systems
  A : PMIOPort  Side=Right
  B : PMIOPort  Port=2  Side=Right
  C : PMIOPort  Port=3  Side=Right
  m : Outport
  wires:
  Generator Measures/3(wm) -> Diesel Engine Governor/2(w (pu))
  Generator Measures/2(Vt) -> Excitation System/2
  Selected Measurements/1(sm) -> m/1, [GenM]
  Synchronous Machine/1 -> Generator Measures/1(m), Selected Measurements/1(m)
  Ground/1 -> Excitation System/4
  Generator Measures/1(Ifd) -> Excitation System/3
  Diesel Engine Governor/1(Pmec (pu)) -> Synchronous Machine/1
  Excitation System/1 -> Synchronous Machine/2
  [GenM] -> Automatic Generator Controls/3(GenM)
  PQwv_ref/1 -> Automatic Generator Controls/2(PQwv_ref)
  Mode/1 -> Automatic Generator Controls/1(Mode)
  Automatic Generator Controls/1(wref) -> Diesel Engine Governor/1(wref (pu))
  Automatic Generator Controls/2(vref) -> Excitation System/1
  connections:
  Synchronous Machine/RConn1 -- Shunt/LConn1 -- A/RConn1
  Synchronous Machine/RConn3 -- Shunt/LConn3 -- C/RConn1
  Synchronous Machine/RConn2 -- Shunt/LConn2 -- B/RConn1

== system exampleMicrogridLibrary/Diesel Generator (GOV, AVR only)/Generator Measures ==
  m : Inport
  Bus Selector : BusSelector  OutputSignals="dq0 components.Stator voltage  vq (pu),dq0 components.Stator voltage  vd (pu)"  OutputAsBus=on
  Bus Selector1 : BusSelector  OutputSignals="Mechanical.Rotor speed  wm  (pu),dq0 components.Field current  ifd (pu)"
  Fcn1 : Fcn  Expr=sqrt(u(1)^2 + u(2)^2)
  Ifd : Outport
  Vt : Outport  Port=2
  wm : Outport  Port=3
  wires:
  Bus Selector1/1 -> wm/1  "<Rotor speed  wm  (pu)>"
  m/1 -> Bus Selector1/1, Bus Selector/1
  Fcn1/1 -> Vt/1
  Bus Selector/1 -> Fcn1/1
  Bus Selector1/2 -> Ifd/1  "<Field current  ifd (pu)>"

== system exampleMicrogridLibrary/Diesel Generator (GOV, AVR only)/Selected Measurements ==
  m : Inport
  Bus Creator : BusCreator  Inputs=7
  Bus Selector : BusSelector  OutputSignals="Mechanical.Electrical power  Pe (pu),Mechanical.Rotor speed  wm  (pu),Output active power   Peo (pu),Output reactive power  Qeo (pu)"
  to W : Gain  Gain=Pn
  to W1 : Gain  Gain=Pn
  to W2 : Gain  Gain=Pn
  sm : Outport
  wires:
  to W2/1 -> Bus Creator/7  "Reactive Power (W)"
  to W1/1 -> Bus Creator/6  "Active Power (W)"
  Bus Selector/2 -> Bus Creator/3  "<Rotor speed  wm  (pu)>"
  Bus Creator/1 -> sm/1
  to W/1 -> Bus Creator/1  "Electrical Power (W)"
  Bus Selector/3 -> Bus Creator/4, to W1/1  "<Output active power   Peo (pu)>"
  Bus Selector/1 -> to W/1, Bus Creator/2  "<Electrical power  Pe (pu)>"
  Bus Selector/4 -> Bus Creator/5, to W2/1  "<Output reactive power  Qeo (pu)>"
  m/1 -> Bus Selector/1

== system exampleMicrogridLibrary/Diesel Generator (Simple Controls)/Continuous ==
  wref (pu) : Inport
  Vref (pu) : Inport  Port=2
  Diesel Engine Governor : spsDieselMotorModel/Diesel Engine Governor  K=29  Tr=[0.01 0.02 0.2]  Ta=[0.25 0.009 0.0384]  Tlim=[0 1.1]  Td=0.024  Pm0=0.84379
  Excitation System : sps_avr/AC1A Excitation System  Tr=20e-3  KaTa=[400 0.02]  VAminmax=[-14.5 14.5]  VRminmax=[-5.43 6.03]  KfTf=[0.03 1.0]  TbTc=[0 0]  KeTe=[1.0 0.80]  Ve12=[4.18 3.14]  SeVe12=[0.10 0.03]  Kd=0.38  Kc=0.20  v0=[1 1.3376]  TsBlock=0
      settings: SourceProductName=Simscape Power Systems  SourceProductBaseCode=PS
  Generator Measures : Subsystem
  Ground : Ground
  Selected Measurements : Subsystem
  Shunt : powerlib/Elements/Three-Phase Parallel RLC Load  LConnTagsString=A|B|C  Configuration=Y (grounded)  NominalVoltage=Vn  Vabc=[1e3 1e3 1e3]  Vabcp=[1e3 1e3 1e3]  NominalFrequency=Fn  UnbalancedPower=off  ActivePower=Pn*0.05  InductivePower=0  CapacitivePower=0  Pabc=[10e3 9e3 11e3]  QLabc=[100 90 110]  QCabc=[100 90 110]  Pabcp=[10e3 9e3 11e3]  QLabcp=[100 90 110]  QCabcp=[100 90 110]  Measurements=None  LoadType=constant Z
  Synchronous Machine : powerlib/Machines/Synchronous Machine pu Standard  PresetModel=No  MechanicalLoad=Mechanical power Pm  ShowDetailedParameters=on  RotorType=Salient-pole  Units=per unit standard parameters  MeasurementBus=off  NominalParameters=[ Pn Vn Fn]  Reactances1=[ 1.81, 0.3, 0.23, 1.76, 0.65, 0.25, 0.15 ]  Reactances2="[ 1.305, 0.296, 0.252, 0.474,  0.243,  0.18 ]"  dAxisTimeConstants=Open-circuit  qAxisTimeConstants=Short-circuit  TimeConstants1="[ 4.4849  0.0681  0.1  ]"  TimeConstants2=[ 8.0, 0.03, 1.0, 0.07 ]  TimeConstants3="[  4.49  0.0681  0.0513  ]"  TimeConstants4=[ 8.0, 0.03, 0.3371, 0.0295 ]  TimeConstants5=[ 1.01, 0.053, 0.1 ]  TimeConstants6=[ 1.3201, 0.023, 1.0, 0.07 ]  TimeConstants7=[0.012 0.003 0.003]  TimeConstants8=[ 1.3201, 0.0231, 0.3371, 0.0295 ]  StatorResistance=0.003  Mechanical=[3.7 0 1 ]  PolePairs=20  InitialConditions=[0 -68.3001 0.841667 0.841667 0.841667 4.44859e-14 -120 120 1.3376]  SetSaturation=off  Saturation=[0.6404,0.7127,0.8441,0.9214,0.9956,1.082,1.19,1.316,1.457;0.7,0.7698,0.8872,0.9466,0.9969,1.046,1.1,1.151,1.201]  LoadFlowParameters=[1,0,0,0,0]  TsPowergui=0  TsBlock=-1  IterativeModel=Trapezoidal non iterative  IterativeDiscreteModel=Trapezoidal non iterative  BusType=swing  Pref=Pn*P0  Qref=0  Qmin=-inf  Qmax=inf  PLF=0  QLF=0
      settings: SourceProductName=Simscape Power Systems
  A : PMIOPort  Side=Right
  B : PMIOPort  Port=2  Side=Right
  C : PMIOPort  Port=3  Side=Right
  m : Outport
  wires:
  Generator Measures/3(wm) -> Diesel Engine Governor/2
  Vref (pu)/1 -> Excitation System/1
  Selected Measurements/1(sm) -> m/1
  Synchronous Machine/1 -> Generator Measures/1(m), Selected Measurements/1(m)
  Ground/1 -> Excitation System/4
  Generator Measures/1(Ifd) -> Excitation System/3
  Diesel Engine Governor/1 -> Synchronous Machine/1
  wref (pu)/1 -> Diesel Engine Governor/1
  Excitation System/1 -> Synchronous Machine/2
  Generator Measures/2(Vt) -> Excitation System/2
  connections:
  Synchronous Machine/RConn1 -- Shunt/LConn1 -- A/RConn1
  Synchronous Machine/RConn3 -- Shunt/LConn3 -- C/RConn1
  Synchronous Machine/RConn2 -- Shunt/LConn2 -- B/RConn1

== system exampleMicrogridLibrary/Diesel Generator (Simple Controls)/Discrete ==
  wref (pu) : Inport
  Vref (pu) : Inport  Port=2
  Diesel Engine Governor : Subsystem  mask(Diesel Engine & Governor){K=29, Tr=[0.01 0.02 0.2], Ta=[0.25 0.009 0.0384], Tlim=[0 1.1], Td=0.024, Pm0=0.84379, Ts=Ts}
      mask prompts: K "Regulator gain K:"; Tr "Regulator time constants [T1 T2 T3 ] (s) :"; Ta "Actuator time constants [T4 T5 T6] (s) :"; Tlim "Torque limits [Tmin Tmax] (pu) :"; Td "Engine time delay Td (s) :"; Pm0 "Initial value of mechanical power  Pm0 (pu) :"; Ts "Sample Time (s)"
      mask help:
      | This block implements a diesel engine and governor system:
      | 1st and 2nd inputs: Desired and actual speed (pu)
      | Output: Diesel engine mechanical power.Motor inertia should be combined with generator.
      | Controller transfer function:
      |      Hc=K.(1+T3.s)/(1+T1.s+T1.T2.s^2)
      | Actuator transfer function :
      |      Ha= (1+T4.s) / [ (s (1+T5.s)(1+T6.s) ]
      | Motor :
      |      Time delay Td
      |
      | (See reference in Tutorial Session 5)
  Excitation System : sps_avr/AC1A Excitation System  Tr=20e-3  KaTa=[400 0.02]  VAminmax=[-14.5 14.5]  VRminmax=[-5.43 6.03]  KfTf=[0.03 1.0]  TbTc=[0 0]  KeTe=[1.0 0.80]  Ve12=[4.18 3.14]  SeVe12=[0.10 0.03]  Kd=0.38  Kc=0.20  v0=[1 1.3376]  TsBlock=Ts
      settings: SourceProductName=Simscape Power Systems  SourceProductBaseCode=PS
  Generator Measures : Subsystem
  Ground : Ground
  Selected Measurements : Subsystem
  Shunt : powerlib/Elements/Three-Phase Parallel RLC Load  LConnTagsString=A|B|C  Configuration=Y (grounded)  NominalVoltage=Vn  Vabc=[1e3 1e3 1e3]  Vabcp=[1e3 1e3 1e3]  NominalFrequency=Fn  UnbalancedPower=off  ActivePower=Pn*0.05  InductivePower=0  CapacitivePower=0  Pabc=[10e3 9e3 11e3]  QLabc=[100 90 110]  QCabc=[100 90 110]  Pabcp=[10e3 9e3 11e3]  QLabcp=[100 90 110]  QCabcp=[100 90 110]  Measurements=None  LoadType=constant Z
  Synchronous Machine : powerlib/Machines/Synchronous Machine pu Standard  PresetModel=No  MechanicalLoad=Mechanical power Pm  ShowDetailedParameters=on  RotorType=Salient-pole  Units=per unit standard parameters  MeasurementBus=off  NominalParameters=[ Pn Vn Fn]  Reactances1=[ 1.81, 0.3, 0.23, 1.76, 0.65, 0.25, 0.15 ]  Reactances2="[ 1.305, 0.296, 0.252, 0.474,  0.243,  0.18 ]"  dAxisTimeConstants=Open-circuit  qAxisTimeConstants=Short-circuit  TimeConstants1="[ 4.4849  0.0681  0.1  ]"  TimeConstants2=[ 8.0, 0.03, 1.0, 0.07 ]  TimeConstants3="[  4.49  0.0681  0.0513  ]"  TimeConstants4=[ 8.0, 0.03, 0.3371, 0.0295 ]  TimeConstants5=[ 1.01, 0.053, 0.1 ]  TimeConstants6=[ 1.3201, 0.023, 1.0, 0.07 ]  TimeConstants7=[0.012 0.003 0.003]  TimeConstants8=[ 1.3201, 0.0231, 0.3371, 0.0295 ]  StatorResistance=0.003  Mechanical=[3.7 0 1 ]  PolePairs=20  InitialConditions=[0 -68.3001 0.841667 0.841667 0.841667 4.44859e-14 -120 120 1.3376]  SetSaturation=off  Saturation=[0.6404,0.7127,0.8441,0.9214,0.9956,1.082,1.19,1.316,1.457;0.7,0.7698,0.8872,0.9466,0.9969,1.046,1.1,1.151,1.201]  LoadFlowParameters=[1,0,0,0,0]  TsPowergui=0  TsBlock=Ts  IterativeModel=Trapezoidal non iterative  IterativeDiscreteModel=Trapezoidal non iterative  BusType=PQ  Pref=Pn*P0  Qref=0  Qmin=-inf  Qmax=inf  PLF=0  QLF=0
      settings: SourceProductName=Simscape Power Systems
  A : PMIOPort  Side=Right
  B : PMIOPort  Port=2  Side=Right
  C : PMIOPort  Port=3  Side=Right
  m : Outport
  wires:
  Excitation System/1 -> Synchronous Machine/2
  wref (pu)/1 -> Diesel Engine Governor/1(wref (pu))
  Diesel Engine Governor/1(Pmec (pu)) -> Synchronous Machine/1
  Generator Measures/1(Ifd) -> Excitation System/3
  Ground/1 -> Excitation System/4
  Synchronous Machine/1 -> Selected Measurements/1(m), Generator Measures/1(m)
  Selected Measurements/1(sm) -> m/1
  Generator Measures/2(Vt) -> Excitation System/2
  Vref (pu)/1 -> Excitation System/1
  Generator Measures/3(wm) -> Diesel Engine Governor/2(w (pu))
  connections:
  Synchronous Machine/RConn2 -- Shunt/LConn2 -- B/RConn1
  Synchronous Machine/RConn3 -- Shunt/LConn3 -- C/RConn1
  Synchronous Machine/RConn1 -- Shunt/LConn1 -- A/RConn1

== system exampleMicrogridLibrary/Energy Storage (PQ Model)/Charge Limits ==
  SOC (%) : Inport
  Pin : Inport  Port=2
  Qin : Inport  Port=3
  Overcharge Check : Subsystem
  Undercharge Check : Subsystem
  Pbatt : Outport
  Qbatt : Outport  Port=2
  wires:
  SOC (%)/1 -> Overcharge Check/1(SOC (%)), Undercharge Check/1(SOC (%))
  Undercharge Check/2(Qout) -> Qbatt/1
  Pin/1 -> Overcharge Check/2(Pin)
  Overcharge Check/1(Pout) -> Undercharge Check/2(Pin)
  Qin/1 -> Overcharge Check/3(Qin)
  Undercharge Check/1(Pout) -> Pbatt/1  "Pbatt"
  Overcharge Check/2(Qout) -> Undercharge Check/3(Qin)

== system exampleMicrogridLibrary/Energy Storage (PQ Model)/Disable PQ Source if VF Control ==
  Pdes : Inport
  Mode : Inport  Port=2
  Qdes : Inport  Port=3
  Constant : Constant  Value=0
  Constant1 : Constant  Value=0
  Switch2 : Switch  Criteria=u2 > Threshold
  Switch3 : Switch  Criteria=u2 > Threshold
  Pbatt : Outport
  Qbatt : Outport  Port=2
  wires:
  Mode/1 -> Switch3/2, Switch2/2
  Pdes/1 -> Switch2/1
  Switch2/1 -> Pbatt/1
  Constant1/1 -> Switch3/3
  Switch3/1 -> Qbatt/1
  Constant/1 -> Switch2/3
  Qdes/1 -> Switch3/1

== system exampleMicrogridLibrary/Energy Storage (PQ Model)/Power Measures ==
  EMT : Subsystem  VariantControl=EMT
  Phasor : Subsystem  VariantControl=Phasor
  A : PMIOPort  Side=Left
  a : PMIOPort  Port=2  Side=Right
  B : PMIOPort  Port=3  Side=Left
  b : PMIOPort  Port=4  Side=Right
  C : PMIOPort  Port=5  Side=Left
  c : PMIOPort  Port=6  Side=Right
  P : Outport
  Q : Outport  Port=2

== system exampleMicrogridLibrary/Energy Storage (PQ Model)/Reactive Power Capability ==
  Pin : Inport
  Qin : Inport  Port=2
  Constant : Constant  Value=Pnom
  Math Function : Math  Operator=square  SaturateOnIntegerOverflow=on
  Math Function1 : Math  Operator=square  SaturateOnIntegerOverflow=on
  Saturation Dynamic : simulink/Discontinuities/Saturation Dynamic  OutMin=[]  OutMax=[]  OutDataTypeStr=Inherit: Same as second input  OutDataType=fixdt(1, 16)  OutScaling=2^-10  DoSatur=off
  Sqrt : Sqrt  SaturateOnIntegerOverflow=on
  Sum : Sum  Inputs=-+|
  Unary Minus : UnaryMinus
  Qout : Outport
  wires:
  Sqrt/1 -> Saturation Dynamic/1, Unary Minus/1
  Math Function1/1 -> Sum/1
  Math Function/1 -> Sum/2
  Constant/1 -> Math Function/1
  Sum/1 -> Sqrt/1
  Unary Minus/1 -> Saturation Dynamic/3
  Saturation Dynamic/1 -> Qout/1
  Pin/1 -> Math Function1/1
  Qin/1 -> Saturation Dynamic/2

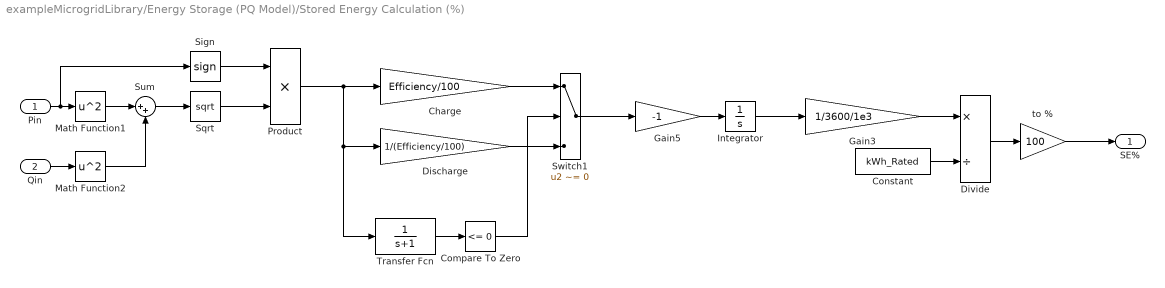
== system exampleMicrogridLibrary/Energy Storage (PQ Model)/Stored Energy Calculation (%) ==
  Pin : Inport
  Qin : Inport  Port=2
  Charge : Gain  Gain=Efficiency/100
  Compare To Zero : simulink/Logic and Bit Operations/Compare To Zero  relop=<=  OutDataTypeStr=boolean
  Constant : Constant  Value=kWh_Rated
  Discharge : Gain  Gain=1/(Efficiency/100)
  Divide : Product  Inputs=*/
  Gain3 : Gain  Gain=1/3600/1e3
  Gain5 : Gain  Gain=-1
  Integrator : Integrator  InitialCondition=(Initial_kWh_pc/100)*kWh_Rated*3600*1e3
  Math Function1 : Math  Operator=square  SaturateOnIntegerOverflow=on
  Math Function2 : Math  Operator=square  SaturateOnIntegerOverflow=on
  Product : Product
  Sign : Signum
  Sqrt : Sqrt  SaturateOnIntegerOverflow=on
  Sum : Sum  Inputs=|++
  Switch1 : Switch  Criteria=u2 ~= 0
  Transfer Fcn : TransferFcn  Denominator=[1 1]
  to % : Gain  Gain=100
  SE% : Outport
  wires:
  Sign/1 -> Product/1
  Sqrt/1 -> Product/2
  Sum/1 -> Sqrt/1
  Math Function2/1 -> Sum/2
  Math Function1/1 -> Sum/1
  Qin/1 -> Math Function2/1
  Pin/1 -> Math Function1/1, Sign/1
  Product/1 -> Transfer Fcn/1, Discharge/1, Charge/1
  Discharge/1 -> Switch1/3
  Gain5/1 -> Integrator/1
  to %/1 -> SE%/1
  Transfer Fcn/1 -> Compare To Zero/1
  Switch1/1 -> Gain5/1
  Gain3/1 -> Divide/1
  Constant/1 -> Divide/2
  Charge/1 -> Switch1/1
  Divide/1 -> to %/1
  Compare To Zero/1 -> Switch1/2
  Integrator/1 -> Gain3/1

== system exampleMicrogridLibrary/Fault /Fault A ==
  c : Inport
  Breaker : PMComponent  PhysicalDomain=powersysdomain  LeftPortType=p1  RightPortType=p1  LConnTagsString=a  RConnTagsString=__new0  mask(InnerPowersysBlock){}
  ITAIL : Terminator
  Model : Subsystem
  1 : PMIOPort  Side=Left
  2 : PMIOPort  Port=2  Side=Right
  tag scope: LibraryTag=global
  wires:
  [LibraryTag] -> ITAIL/1
  Model/1(gate) -> [LibraryTag]
  [LibraryTag] -> Model/2(Uswitch)
  c/1 -> Model/1("gate ")
  connections:
  1/RConn1 -- Breaker/LConn1
  2/RConn1 -- Breaker/RConn1

== system exampleMicrogridLibrary/Fault /Fault B ==
  c : Inport
  Breaker : PMComponent  PhysicalDomain=powersysdomain  LeftPortType=p1  RightPortType=p1  LConnTagsString=a  RConnTagsString=__new0  mask(InnerPowersysBlock){}
  ITAIL : Terminator
  Model : Subsystem
  1 : PMIOPort  Side=Left
  2 : PMIOPort  Port=2  Side=Right
  tag scope: LibraryTag=global
  wires:
  [LibraryTag] -> ITAIL/1
  Model/1(gate) -> [LibraryTag]
  [LibraryTag] -> Model/2(Uswitch)
  c/1 -> Model/1("gate ")
  connections:
  1/RConn1 -- Breaker/LConn1
  2/RConn1 -- Breaker/RConn1
